simulink model "sampleModel190"  (R2021b)
settings: Solver=VariableStepAuto  StartTime=0.0  StopTime=10.0  RelTol=1e-3
undefined symbols (not defined in the file or in its folder): magnitude
libraries: simulink x7, slpidlib x1
settings Model: Creator=user  LastModifiedBy=user

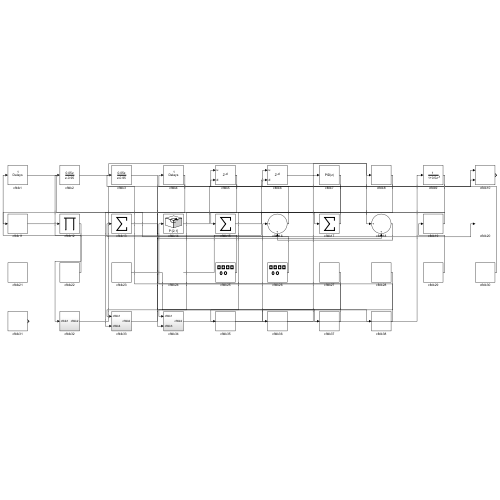
[thumbnail: Simulink's stored preview of the top-level diagram]
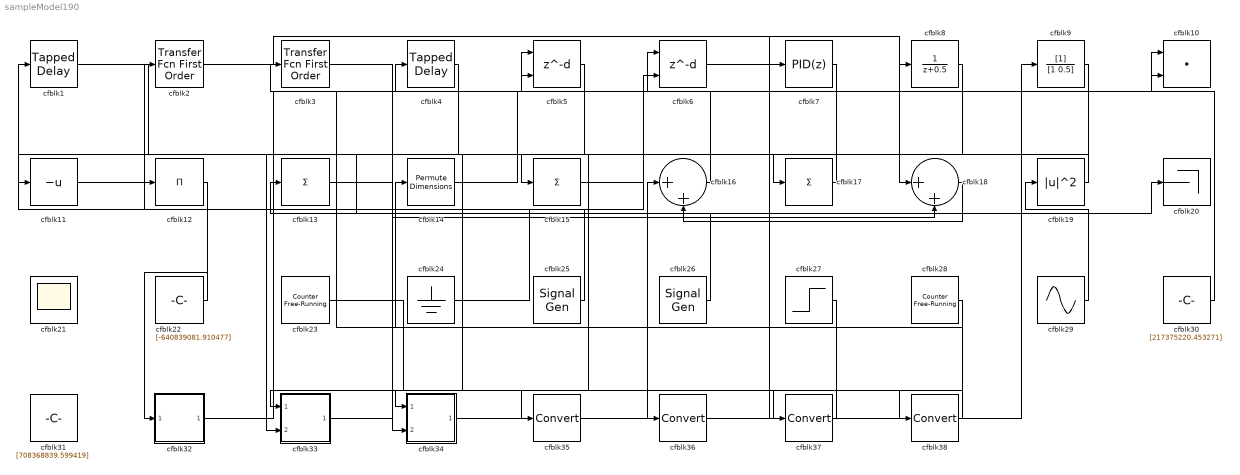
== system sampleModel190 ==
  cfblk1 : simulink/Discrete/Tapped Delay  vinit=0.0  samptime=-1  NumDelays=1  DelayOrder=Oldest  includeCurrent=off
  cfblk10 : DotProduct  InputSameDT=on  OutDataTypeStr=Inherit: Inherit via internal rule
  cfblk11 : UnaryMinus
  cfblk12 : Product  Inputs=*
  cfblk13 : Sum  Inputs=+
  cfblk14 : PermuteDimensions
  cfblk15 : Sum  Inputs=+
  cfblk16 : Sum  Inputs=|++
  cfblk17 : Sum  Inputs=+
  cfblk18 : Sum  Inputs=|++
  cfblk19 : Math  Operator=magnitude^2  SaturateOnIntegerOverflow=on
  cfblk2 : simulink/Discrete/Transfer Fcn First Order  PoleZ=0.95  ICPrevOutput=0.0  DoSatur=off
  cfblk20 : Terminator
  cfblk21 : Scope
      settings: Floating=on
  cfblk22 : Constant  Value=[-640839081.910477]  SampleTime=1
  cfblk23 : simulink/Sources/Counter Free-Running  NumBits=[46.000000]  tsamp=-1
  cfblk24 : Ground
  cfblk25 : SignalGenerator  WaveForm=sawtooth  Amplitude=[109230491.198578]
  cfblk26 : SignalGenerator  Amplitude=[577572685.866582]
  cfblk27 : Step  Time=[26.000000]  Before=[366964797.184170]  After=[-51553592.084691]  SampleTime=0
  cfblk28 : simulink/Sources/Counter Free-Running  NumBits=[39.000000]  tsamp=-1
  cfblk29 : Sin  Amplitude=[27266409.032489]  Bias=[398070011.647885]  SampleTime=0
  cfblk3 : simulink/Discrete/Transfer Fcn First Order  PoleZ=0.95  ICPrevOutput=0.0  DoSatur=off
  cfblk30 : Constant  Value=[217375220.453271]  SampleTime=1
  cfblk31 : Constant  Value=[708368839.599419]  SampleTime=1
  cfblk32 : Subsystem
  cfblk33 : Subsystem
  cfblk34 : Subsystem
  cfblk{35..38} (4 alike) : DataTypeConversion
  cfblk4 : simulink/Discrete/Tapped Delay  vinit=0.0  samptime=-1  NumDelays=1  DelayOrder=Oldest  includeCurrent=off
  cfblk5 : Delay  DelayLengthSource=Input port  SampleTime=1
      settings: InputPortMap=u0,p1
  cfblk6 : Delay  DelayLengthSource=Input port  SampleTime=1
      settings: InputPortMap=u0,p1
  cfblk7 : slpidlib/PID Controller  Controller=PID  Form=Parallel  TimeDomain=Discrete-time  UseExternalTs=off  SampleTime=1  IntegratorMethod=Forward Euler  FilterMethod=Forward Euler  ControllerParametersSource=internal  P=1  I=1  D=0  UseFilter=on  N=100  TunerSelectOption=Transfer Function Based (PID Tuner App)  InitialConditionSource=internal  InitialConditionForIntegrator=0  InitialConditionForFilter=0  DifferentiatorICPrevScaledInput=0  ExternalReset=none  TrackingMode=off  Kt=1  LimitOutput=off  SatLimitsSource=internal  UpperSaturationLimit=inf  LowerSaturationLimit=-inf  LinearizeAsGain=off  AntiWindupMode=none  Kb=1  POutMin=[]  POutMax=[]  IOutMin=[]  IOutMax=[]  DOutMin=[]  DOutMax=[]  NOutMin=[]  NOutMax=[]  SumOutMin=[]  SumOutMax=[]  SaturationOutMin=[]  SaturationOutMax=[]  PParamMin=[]  PParamMax=[]  IParamMin=[]  IParamMax=[]  DParamMin=[]  DParamMax=[]  NParamMin=[]  NParamMax=[]  KbParamMin=[]  KbParamMax=[]  KtParamMin=[]  KtParamMax=[]  KbOutMin=[]  KbOutMax=[]  KtOutMin=[]  KtOutMax=[]  IntegratorOutMin=[]  IntegratorOutMax=[]  FilterOutMin=[]  FilterOutMax=[]  SumI1OutMin=[]  SumI1OutMax=[]  SumI2OutMin=[]  SumI2OutMax=[]  SumI3OutMin=[]  SumI3OutMax=[]  SumI4OutMin=[]  SumI4OutMax=[]  SumDOutMin=[]  SumDOutMax=[]  DifferentiatorOutMin=[]  DifferentiatorOutMax=[]  FilterDiffOutCoefMin=[]  FilterDiffOutCoefMax=[]  ReciprocalOutMin=[]  ReciprocalOutMax=[]  SumDenOutMin=[]  SumDenOutMax=[]  SumNumOutMin=[]  SumNumOutMax=[]  DivideOutMin=[]  DivideOutMax=[]  UdiffTsProdOutMin=[]  UdiffTsProdOutMax=[]  NTsProdOutMin=[]  NTsProdOutMax=[]  UintegralTsProdOutMin=[]  UintegralTsProdOutMax=[]  UngainTsProdOutMin=[]  UngainTsProdOutMax=[]  IntegratorContinuousStateAttributes=''  IntegratorStateMustResolveToSignalObject=off  IntegratorRTWStateStorageClass=Auto  FilterContinuousStateAttributes=''  FilterStateMustResolveToSignalObject=off  FilterRTWStateStorageClass=Auto  ParallelPVariant=InternalParameters  IdealPVariant=Disabled  IVariant=InternalParameters  DVariant=InternalParameters  IntegratorVariant=Discrete  SatVariant=Disabled  AWVariant=Passthrough  PCopyVariant=Disabled  TRVariant=Disabled  FdbkBlocksVariant=Forward  IdealPFdbkVariant=Disabled  SatFdbkVariant=Disabled  DerivativeFilterVariant=ForwardEulerFilter  NVariant=InternalParameters  NCopyVariant=Disabled  FilterICVariant=InternalICsFilter  IntegratorICVariant=InternalICs  ExternalResetVariant=Disabled  TRSumVariant=Passthrough  SumFdbkVariant=Disabled  SumVariant=Sum_PID  TsampFilterVariant=InternalTs  TsampNgainVariant=Passthrough  TsampIntegralVariant=Passthrough  ExternalSaturationOutDataTypeStr=Inherit: Same as second input
  cfblk8 : DiscreteTransferFcn  SampleTime=1
  cfblk9 : DiscreteFilter  SampleTime=1
  wires:
  cfblk7/1 -> cfblk15/1
  cfblk12/1 -> cfblk32/1(cfblk1)
  cfblk2/1 -> cfblk18/1
  cfblk1/1 -> cfblk20/1
  cfblk25/1 -> cfblk2/1
  cfblk34/1(cfblk2) -> cfblk16/1
  cfblk11/1 -> cfblk12/1
  cfblk22/1 -> cfblk1/1
  cfblk17/1 -> cfblk5/1
  cfblk32/1(cfblk2) -> cfblk5/2
  cfblk29/1 -> cfblk19/1
  cfblk5/1 -> cfblk34/1(cfblk1)
  cfblk16/1 -> cfblk4/1
  cfblk26/1 -> cfblk13/1
  cfblk27/1 -> cfblk33/1(cfblk1)
  cfblk13/1 -> cfblk18/2
  cfblk30/1 -> cfblk6/1
  cfblk24/1 -> cfblk6/2
  cfblk18/1 -> cfblk16/2
  cfblk15/1 -> cfblk17/1
  cfblk8/1 -> cfblk34/2(cfblk3)
  cfblk4/1 -> cfblk33/2(cfblk4)
  cfblk6/1 -> cfblk8/1
  cfblk19/1 -> cfblk11/1
  cfblk14/1 -> cfblk10/1
  cfblk33/1(cfblk2) -> cfblk10/2
  cfblk9/1 -> cfblk35/1
  cfblk35/1 -> cfblk7/1
  cfblk28/1 -> cfblk36/1
  cfblk36/1 -> cfblk9/1
  cfblk3/1 -> cfblk37/1
  cfblk37/1 -> cfblk14/1
  cfblk23/1 -> cfblk38/1
  cfblk38/1 -> cfblk3/1

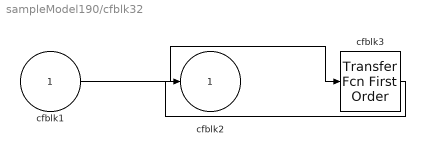
== system sampleModel190/cfblk32 ==
  cfblk1 : Inport
  cfblk3 : simulink/Discrete/Transfer Fcn First Order  PoleZ=0.95  ICPrevOutput=0.0  DoSatur=off
  cfblk2 : Outport
  wires:
  cfblk1/1 -> cfblk3/1
  cfblk3/1 -> cfblk2/1

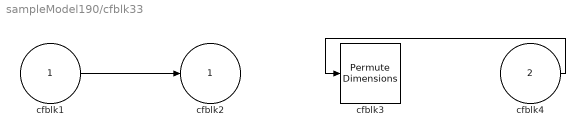
== system sampleModel190/cfblk33 ==
  cfblk1 : Inport
  cfblk4 : Inport  Port=2
  cfblk3 : PermuteDimensions
  cfblk2 : Outport
  wires:
  cfblk1/1 -> cfblk2/1
  cfblk4/1 -> cfblk3/1

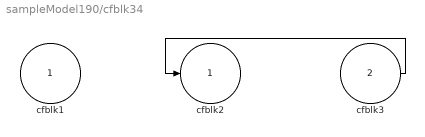
== system sampleModel190/cfblk34 ==
  cfblk1 : Inport
  cfblk3 : Inport  Port=2
  cfblk2 : Outport
  wires:
  cfblk3/1 -> cfblk2/1
